simulink model "task2b_j"  (R2019a)
settings: Solver=VariableStepAuto  StartTime=0.0  StopTime=10.0  RelTol=1e-3
settings Model: Creator=Artem  LastModifiedBy=Artem

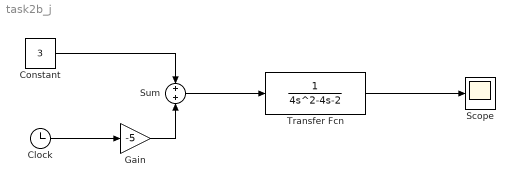
== system task2b_j ==
  Clock : Clock
  Constant : Constant  Value=3
  Gain : Gain  Gain=-5
  Scope : Scope
  Sum : Sum
  Transfer Fcn : TransferFcn  Denominator=[4 -4 -2]
  wires:
  Clock/1 -> Gain/1
  Gain/1 -> Sum/2
  Constant/1 -> Sum/1
  Transfer Fcn/1 -> Scope/1
  Sum/1 -> Transfer Fcn/1
